simulink model "bldc_model"  (R2018b)
settings: Solver=VariableStepAuto  StartTime=0.0  StopTime=10.0  RelTol=1e-3
settings Model: Creator=TUAN HUA  LastModifiedBy=TUAN HUA

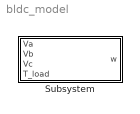
== system bldc_model ==
  Subsystem : Subsystem  mask{L=0, R=0, J=0, B=0, p=0}
      mask prompts: L "Armature self-inductance, L(H)"; R "Armature resistance, R (Ohm)"; J "Motor inertia"; B "Motor damping"; p "Number of pole"

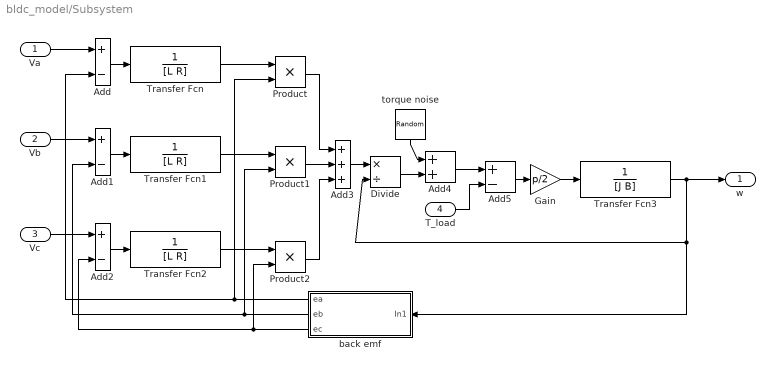
== system bldc_model/Subsystem ==
  Va : Inport
  Vb : Inport  Port=2
  Vc : Inport  Port=3
  T_load : Inport  Port=4
  Add{,1..2,5} (4 alike) : Sum  Inputs=+-
  Add3 : Sum  Inputs=+++
  Add4 : Sum
  Divide : Product  Inputs=*/
  Gain : Gain  Gain=p/2
  Product : Product
  Product1 : Product
  Product2 : Product
  Transfer Fcn : TransferFcn  Denominator=[L R]
  Transfer Fcn1 : TransferFcn  Denominator=[L R]
  Transfer Fcn2 : TransferFcn  Denominator=[L R]
  Transfer Fcn3 : TransferFcn  Denominator=[J B]
  back emf : Subsystem
  torque noise : RandomNumber  Variance=0.01  SampleTime=0.1
  w : Outport
  wires:
  Va/1 -> Add/1
  Vb/1 -> Add1/1
  Add/1 -> Transfer Fcn/1
  Add1/1 -> Transfer Fcn1/1
  Add2/1 -> Transfer Fcn2/1
  Vc/1 -> Add2/1
  back emf/1(ea) -> Product/2, Add/2
  back emf/2(eb) -> Product1/2, Add1/2
  back emf/3(ec) -> Product2/2, Add2/2
  Transfer Fcn/1 -> Product/1
  Transfer Fcn1/1 -> Product1/1
  Transfer Fcn2/1 -> Product2/1
  Product/1 -> Add3/1
  Product1/1 -> Add3/2
  Product2/1 -> Add3/3
  Add3/1 -> Divide/1
  Divide/1 -> Add4/2
  torque noise/1 -> Add4/1
  Add4/1 -> Add5/1
  T_load/1 -> Add5/2
  Add5/1 -> Gain/1
  Gain/1 -> Transfer Fcn3/1
  Transfer Fcn3/1 -> back emf/1(In1), Divide/2, w/1

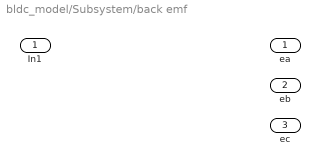
== system bldc_model/Subsystem/back emf ==
  In1 : Inport
  ea : Outport
  eb : Outport  Port=2
  ec : Outport  Port=3
